simulink model "gm_untitled"  (R2020a)
settings: Solver=FixedStepDiscrete  StartTime=0.0  StopTime=10.0  RelTol=1e-3
settings Model: Creator=Mahsa  LastModifiedBy=Mahsa
settings OptimizationCC: BlockReduction=off  ConditionallyExecuteInputs=off  DefaultParameterBehavior=Inlined
settings DebuggingCC: AlgebraicLoopMsg=error  InheritedTsInSrcMsg=none  SingleTaskRateTransMsg=error
settings HardwareCC: ProdBitPerPointer=32  ProdBitPerSizeT=32  ProdBitPerPtrDiffT=32  ProdLargestAtomicFloat=None  ProdIntDivRoundTo=Undefined  ProdEndianess=Unspecified  ProdWordSize=32  ProdHWDeviceType=ASIC/FPGA->ASIC/FPGA  TargetBitPerPointer=64  TargetBitPerSizeT=64  TargetBitPerPtrDiffT=64  TargetLongLongMode=on  TargetIntDivRoundTo=Zero  TargetEndianess=LittleEndian  TargetWordSize=64  TargetHWDeviceType=Custom Processor->MATLAB Host Computer  ProdEqTarget=off

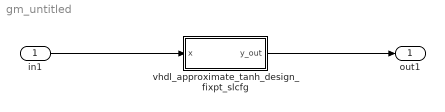
== system gm_untitled ==
  in1 : Inport  OutDataTypeStr=fixdt(1, 14, 10)  PortDimensions=[1 126]  SampleTime=0.2
  vhdl_approximate_tanh_design_fixpt_slcfg : Subsystem
  out1 : Outport
  wires:
  in1/1 -> vhdl_approximate_tanh_design_fixpt_slcfg/1(x)
  vhdl_approximate_tanh_design_fixpt_slcfg/1(y_out) -> out1/1

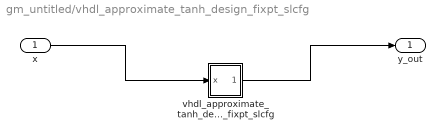
== system gm_untitled/vhdl_approximate_tanh_design_fixpt_slcfg ==
  x : Inport  OutDataTypeStr=fixdt(1, 14, 10)  PortDimensions=[1 126]  SampleTime=0.2
  vhdl_approximate_tanh_design_fixpt_slcfg : MATLAB Function  TreatAsAtomicUnit=on
  y_out : Outport
  wires:
  x/1 -> vhdl_approximate_tanh_design_fixpt_slcfg/1(x)
  vhdl_approximate_tanh_design_fixpt_slcfg/1(y_out) -> y_out/1

== matlab function gm_untitled/vhdl_approximate_tanh_design_fixpt_slcfg/vhdl_approximate_tanh_design_fixpt_slcfg ==
  data: x input fixdt('sfix14_En10') size=[1 126 ]; y_out output
%%%%%%%%%%%%%%%%%%%%%%%%%%%%%%%%%%%%%%%%%%%%%%%%%%%%%%%%%%%%%%%%%%%%%%%%%%%%
%                                                                          %
%           Generated by MATLAB 9.8 and Fixed-Point Designer 7.0           %
%                                                                          %
%%%%%%%%%%%%%%%%%%%%%%%%%%%%%%%%%%%%%%%%%%%%%%%%%%%%%%%%%%%%%%%%%%%%%%%%%%%%
%#codegen
function y_out  = vhdl_approximate_tanh_design_fixpt(x)
%   y_out = 1-(2./(power(2,((2.625)*x))+1));
  fm = get_fimath();

  y_out = fi(cordictanh(x), 1, 14, 13, fm);
end


function fm = get_fimath()
	fm = fimath('RoundingMethod', 'Floor',...
	     'OverflowAction', 'Wrap',...
	     'ProductMode','FullPrecision',...
	     'MaxProductWordLength', 128,...
	     'SumMode','FullPrecision',...
	     'MaxSumWordLength', 128);
end
